simulink model "dc_LQR_1"  (R2019a)
settings: Solver=VariableStepAuto  StartTime=0.0  StopTime=10.0  RelTol=1e-3
values from neighbouring files (symbols this model uses):
  A = [0 1 0;0 -b/J K/J;0 -K/L -R/L]    [state_space_control.m]
  B = [0 ; 0 ; 1/L]    [state_space_control.m]
  C = [1  1  0]    [state_space_control.m]
  kk2 = lqr(A,B,Q,R)    [DC_LQR.m]
settings Model: Creator=asus  LastModifiedBy=asus

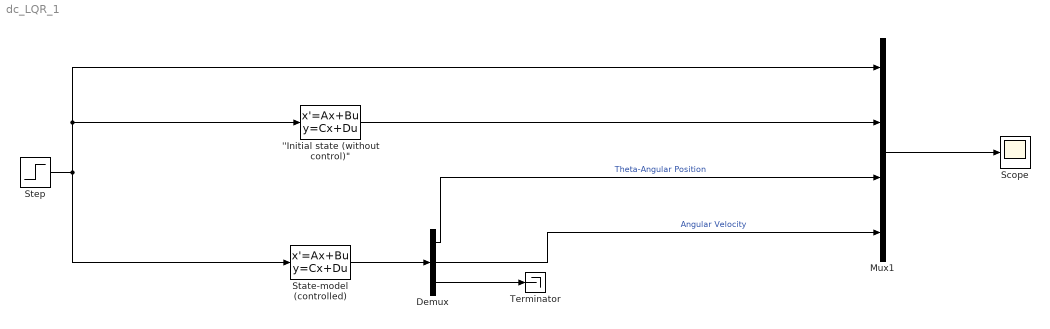
== system dc_LQR_1 ==
  "''Initial state (without control)\"" : StateSpace  A=A  B=B  C=C  D=0  InitialCondition=0
  Demux : Demux  Outputs=3
  Mux1 : Mux
  "Scope " : Scope
  State-model (controlled) : StateSpace  A=A-B*kk2  B=B  C=eye(3)  D=[0;0;0]  InitialCondition=0
  "Step " : Step  SampleTime=0
  Terminator : Terminator
  wires:
  "''Initial state (without control)\""/1 -> Mux1/2
  "Step "/1 -> State-model (controlled)/1, Mux1/1, "''Initial state (without control)\""/1
  Mux1/1 -> "Scope "/1
  Demux/3 -> Terminator/1
  State-model (controlled)/1 -> Demux/1
  Demux/1 -> Mux1/3  "Theta-Angular Position"
  Demux/2 -> Mux1/4  "Angular Velocity"
